simulink model "hodumaru"  (R2023a)
settings: Solver=VariableStepAuto  StartTime=0.0  StopTime=10.0  RelTol=1e-3
undefined symbols (not defined in the file): _NA, Control, DFSW, DSFW, Kill, NeuralCodedData, R_EN, RC, RC_FINAL, Spike
(part 2 of 2)

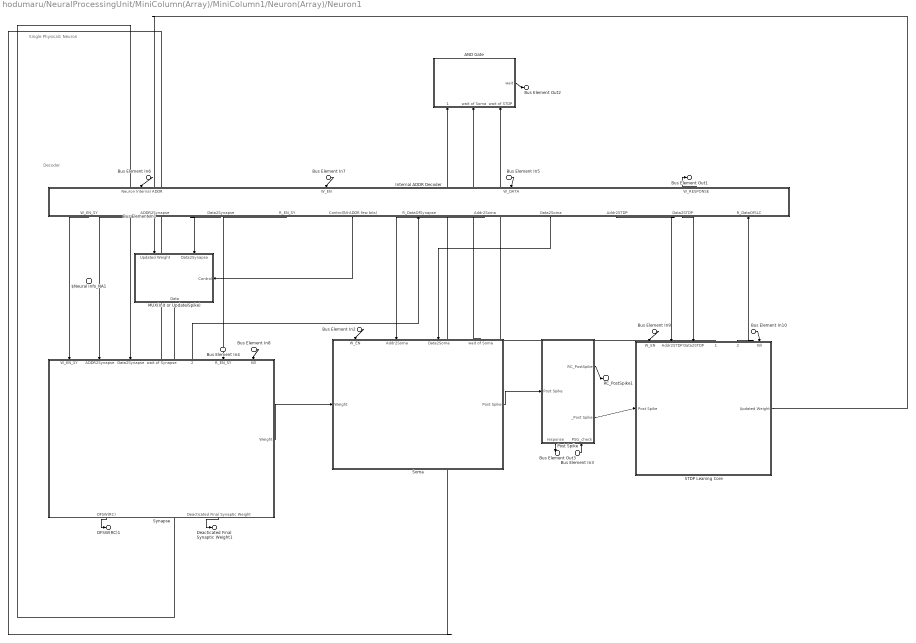
== system hodumaru/NeuralProcessingUnit/MiniColumn(Array)/MiniColumn1/Neuron(Array)/Neuron1 ==
  note: Decoder
  note: Single Physical1 Neuron
  Bus Element In3 : Inport  PortName=PSG_check
  Bus Element In1 : Inport  Port=2  PortName=#Neuron
  Bus Element In6 : Inport  Port=3  PortName=Neuron ADDR
  Bus Element In5 : Inport  Port=4  PortName=W_DATA
  Bus Element In4 : Inport  Port=5  PortName=R_EN
  Bus Element In2 : Inport  Port=6  PortName=W_EN
  Bus Element In7 : Inport  Port=6  PortName=W_EN
  Bus Element In9 : Inport  Port=6  PortName=W_EN
  Bus Element In8 : Inport  Port=7  PortName=Kill
  Bus Element In10 : Inport  Port=7  PortName=Kill
  $Neural Info_NA1 : Inport  Port=8  PortName=$Neural Info_NA
  AND Gate : Subsystem
      settings: PortSchema="{\"entries\":[{\"content\":{\"headerSize\":26,\"margin\":15,\"minimumSpacing\":25,\"sides\":[{\"content\":{},\"type\":\"ConnectorPlacement.EquallySpacedRectSide\",\"uuid\":\"ebe87d50-b34c-4144-bb21-1b9f3994f650\"},{\"content\":{\"connectorIds\":[\"Out1\"],\"side\":\"RIGHT\"},\"type\":\"ConnectorPlacement.EquallySpacedRectSide\",\"uuid\":\"40dc9e4a-9138-4a47-a8ec-83303fc3d098\"},{\"content\":{\"side\":\"TOP\"},\"type\":\"ConnectorPlacement.EquallySpacedRectSide\",\"uuid\":\"74a947e4-452e-4cf6-9818-6ec720a0f546\"},{\"content\":{\"connectorIds\":[\"In1\",\"In2\",\"In3\"],\"side\":\"BOTTOM\"},\"type\":\"ConnectorPlacement.EquallySpacedRectSide\",\"uuid\":\"c5edbbff-3ec9-45d1-a6e5-9e984b0ebe73\"}]},\"type\":\"ConnectorPlacement.EquallySpacedConnector\",\"uuid\":\"10440d1f-8be4-47e4-a65a-b886e6188624\"}],\"packageUris\":[\"http://schema.mathworks.com/mf0/Connector/R2020b\"],\"version\":\"1.0\"}"
  Internal ADDR Decoder : Subsystem
      settings: PortSchema="{\"entries\":[{\"content\":{\"headerSize\":26,\"margin\":15,\"minimumSpacing\":25,\"sides\":[{\"content\":{},\"type\":\"ConnectorPlacement.EquallySpacedRectSide\",\"uuid\":\"ebe87d50-b34c-4144-bb21-1b9f3994f650\"},{\"content\":{\"side\":\"RIGHT\"},\"type\":\"ConnectorPlacement.EquallySpacedRectSide\",\"uuid\":\"40dc9e4a-9138-4a47-a8ec-83303fc3d098\"},{\"content\":{\"connectorIds\":[\"In3\",\"In4\",\"In5\",\"Out3\"],\"side\":\"TOP\"},\"type\":\"ConnectorPlacement.EquallySpacedRectSide\",\"uuid\":\"74a947e4-452e-4cf6-9818-6ec720a0f546\"},{\"content\":{\"connectorIds\":[\"Out1\",\"Out2\",\"Out7\",\"Out4\",\"Out5\",\"In1\",\"Out6\",\"Out9\",\"Out8\",\"Out10\",\"In2\"],\"side\":\"BOTTOM\"},\"type\":\"ConnectorPlacement.EquallySpacedRectSide\",\"uuid\":\"fe67068d-9de4-4d22-acd2-463b28a86914\"}]},\"type\":\"ConnectorPlacement.EquallySpacedConnector\",\"uuid\":\"10440d1f-8be4-47e4-a65a-b886e6188624\"}],\"packageUris\":[\"http://schema.mathworks.com/mf0/Connector/R2020b\"],\"version\":\"1.0\"}"
  MUX(Init or Update/Spike) : Subsystem
      settings: PortSchema="{\"entries\":[{\"content\":{\"headerSize\":26,\"margin\":15,\"minimumSpacing\":25,\"sides\":[{\"content\":{},\"type\":\"ConnectorPlacement.EquallySpacedRectSide\",\"uuid\":\"ebe87d50-b34c-4144-bb21-1b9f3994f650\"},{\"content\":{\"connectorIds\":[\"In1\"],\"side\":\"RIGHT\"},\"type\":\"ConnectorPlacement.EquallySpacedRectSide\",\"uuid\":\"40dc9e4a-9138-4a47-a8ec-83303fc3d098\"},{\"content\":{\"connectorIds\":[\"In2\",\"In3\"],\"side\":\"TOP\"},\"type\":\"ConnectorPlacement.EquallySpacedRectSide\",\"uuid\":\"74a947e4-452e-4cf6-9818-6ec720a0f546\"},{\"content\":{\"connectorIds\":[\"Out1\"],\"side\":\"BOTTOM\"},\"type\":\"ConnectorPlacement.EquallySpacedRectSide\",\"uuid\":\"02f4fd3e-9a7d-4827-bd38-0642fed45587\"}]},\"type\":\"ConnectorPlacement.EquallySpacedConnector\",\"uuid\":\"10440d1f-8be4-47e4-a65a-b886e6188624\"}],\"packageUris\":[\"http://schema.mathworks.com/mf0/Connector/R2020b\"],\"version\":\"1.0\"}"
  Post Spike : Subsystem
      settings: PortSchema="{\"entries\":[{\"content\":{\"headerSize\":26,\"margin\":15,\"minimumSpacing\":25,\"sides\":[{\"content\":{\"connectorIds\":[\"In2\"]},\"type\":\"ConnectorPlacement.EquallySpacedRectSide\",\"uuid\":\"31e20200-2cb1-4382-9155-e0d85eeb6756\"},{\"content\":{\"connectorIds\":[\"Out2\",\"Out3\"],\"side\":\"RIGHT\"},\"type\":\"ConnectorPlacement.EquallySpacedRectSide\",\"uuid\":\"e7a9e024-b9ad-4463-a43b-85143ff39b21\"},{\"content\":{\"side\":\"TOP\"},\"type\":\"ConnectorPlacement.EquallySpacedRectSide\",\"uuid\":\"8c8eb66f-8faf-4222-8ab7-6c33983befa5\"},{\"content\":{\"connectorIds\":[\"Out1\",\"In1\"],\"side\":\"BOTTOM\"},\"type\":\"ConnectorPlacement.EquallySpacedRectSide\",\"uuid\":\"e8737092-59e1-4792-866d-bcd78d7addfa\"}]},\"type\":\"ConnectorPlacement.EquallySpacedConnector\",\"uuid\":\"7102759c-7f33-40ec-8288-a87a26b0547f\"}],\"packageUris\":[\"http://schema.mathworks.com/mf0/Connector/R2020b\"],\"version\":\"1.0\"}"
  STDP Leaning Core : Subsystem
      settings: PortSchema="{\"entries\":[{\"content\":{\"headerSize\":26,\"margin\":15,\"minimumSpacing\":25,\"sides\":[{\"content\":{\"connectorIds\":[\"In5\"]},\"type\":\"ConnectorPlacement.EquallySpacedRectSide\",\"uuid\":\"08b5c2e0-5e4b-4108-9213-5cb3cfbc2fc7\"},{\"content\":{\"connectorIds\":[\"Out3\"],\"side\":\"RIGHT\"},\"type\":\"ConnectorPlacement.EquallySpacedRectSide\",\"uuid\":\"cef344b6-f3e5-417a-912f-da0044eb54ca\"},{\"content\":{\"connectorIds\":[\"In1\",\"In2\",\"In3\",\"Out1\",\"Out2\",\"In4\"],\"side\":\"TOP\"},\"type\":\"ConnectorPlacement.EquallySpacedRectSide\",\"uuid\":\"0b83641f-e918-4d2c-8db0-09bb563129af\"}]},\"type\":\"ConnectorPlacement.EquallySpacedConnector\",\"uuid\":\"45bfd962-fc80-412c-925f-742c48c6b5c0\"}],\"packageUris\":[\"http://schema.mathworks.com/mf0/Connector/R2020b\"],\"version\":\"1.0\"}"
  Soma : Subsystem
      settings: PortSchema="{\"entries\":[{\"content\":{\"headerSize\":26,\"margin\":15,\"minimumSpacing\":25,\"sides\":[{\"content\":{\"connectorIds\":[\"In4\"]},\"type\":\"ConnectorPlacement.EquallySpacedRectSide\",\"uuid\":\"08b5c2e0-5e4b-4108-9213-5cb3cfbc2fc7\"},{\"content\":{\"connectorIds\":[\"Out2\"],\"side\":\"RIGHT\"},\"type\":\"ConnectorPlacement.EquallySpacedRectSide\",\"uuid\":\"cef344b6-f3e5-417a-912f-da0044eb54ca\"},{\"content\":{\"connectorIds\":[\"In1\",\"In2\",\"In3\",\"Out1\"],\"side\":\"TOP\"},\"type\":\"ConnectorPlacement.EquallySpacedRectSide\",\"uuid\":\"0b83641f-e918-4d2c-8db0-09bb563129af\"}]},\"type\":\"ConnectorPlacement.EquallySpacedConnector\",\"uuid\":\"45bfd962-fc80-412c-925f-742c48c6b5c0\"}],\"packageUris\":[\"http://schema.mathworks.com/mf0/Connector/R2020b\"],\"version\":\"1.0\"}"
  Synapse : Subsystem
      settings: PortSchema="{\"entries\":[{\"content\":{\"headerSize\":26,\"margin\":15,\"minimumSpacing\":25,\"sides\":[{\"content\":{},\"type\":\"ConnectorPlacement.EquallySpacedRectSide\",\"uuid\":\"08b5c2e0-5e4b-4108-9213-5cb3cfbc2fc7\"},{\"content\":{\"connectorIds\":[\"Out3\"],\"side\":\"RIGHT\"},\"type\":\"ConnectorPlacement.EquallySpacedRectSide\",\"uuid\":\"cef344b6-f3e5-417a-912f-da0044eb54ca\"},{\"content\":{\"connectorIds\":[\"In1\",\"In2\",\"In3\",\"Out1\",\"Out2\",\"In4\",\"In5\"],\"side\":\"TOP\"},\"type\":\"ConnectorPlacement.EquallySpacedRectSide\",\"uuid\":\"0b83641f-e918-4d2c-8db0-09bb563129af\"},{\"content\":{\"connectorIds\":[\"Out5\",\"Out4\"],\"side\":\"BOTTOM\"},\"type\":\"ConnectorPlacement.EquallySpacedRectSide\",\"uuid\":\"115d5a97-31cb-4c10-ac03-233646a622a9\"}]},\"type\":\"ConnectorPlacement.EquallySpacedConnector\",\"uuid\":\"45bfd962-fc80-412c-925f-742c48c6b5c0\"}],\"packageUris\":[\"http://schema.mathworks.com/mf0/Connector/R2020b\"],\"version\":\"1.0\"}"
  Bus Element Out3 : Outport  PortName=response
  Bus Element Out2 : Outport  Port=2  PortName=wait
  Bus Element Out1 : Outport  Port=3  PortName=W_RESPONSE
  RC_PostSpike1 : Outport  Port=4  PortName=RC_PostSpike
  Deacticated Final Synaptic Weight1 : Outport  Port=5  PortName=Deacticated Final Synaptic Weight
  DFSW(RC)1 : Outport  Port=6  PortName=DFSW(RC)
  wires:
  Synapse/5(DFSW(RC)) -> DFSW(RC)1/1
  STDP Leaning Core/3(Updated Weight) -> MUX(Init or Update/Spike)/2(Updated Weight)
  Synapse/3(Weight) -> Soma/4(Weight)
  Soma/2(Post Spike) -> Post Spike/2(Post Spike)
  Post Spike/3(_Post Spike) -> STDP Leaning Core/5(Post Spike)
  Synapse/4(Deacticated Final Synaptic Weight) -> Deacticated Final Synaptic Weight1/1
  Post Spike/2(RC_PostSpike) -> RC_PostSpike1/1
  Bus Element In2/1 -> Soma/1(W_EN)
  Bus Element In6/1 -> Internal ADDR Decoder/3(Neuron Internal ADDR)
  Internal ADDR Decoder/7(Data2Synapse) -> MUX(Init or Update/Spike)/3(Data2Synapse)
  Internal ADDR Decoder/9(Data2Soma) -> Soma/3(Data2Soma)
  Internal ADDR Decoder/10(Data2STDP) -> STDP Leaning Core/3(Data2STDP)
  Bus Element In5/1 -> Internal ADDR Decoder/5(W_DATA)
  Bus Element In7/1 -> Internal ADDR Decoder/4(W_EN)
  Internal ADDR Decoder/3(W_RESPONSE) -> Bus Element Out1/1
  Internal ADDR Decoder/2(ADDR2Synapse) -> Synapse/2(ADDR2Synapse)
  Internal ADDR Decoder/6(Addr2Soma) -> Soma/2(Addr2Soma)
  Synapse/2(R_DataOfSynapse) -> Internal ADDR Decoder/1(R_DataOfSynapse)
  STDP Leaning Core/2(R_DataOfSLC) -> Internal ADDR Decoder/2(R_DataOfSLC)
  MUX(Init or Update/Spike)/1(Data) -> Synapse/3(Data2Synapse)
  Bus Element In8/1 -> Synapse/5(Kill)
  Internal ADDR Decoder/5(Control(NI-ADDR few bits)) -> MUX(Init or Update/Spike)/1(Control)
  Synapse/1(wait of Synapse) -> AND Gate/1(wait of Synapse)
  Soma/1(wait of Soma) -> AND Gate/2(wait of Soma)
  STDP Leaning Core/1(wait of STDP) -> AND Gate/3(wait of STDP)
  AND Gate/1(wait) -> Bus Element Out2/1
  Internal ADDR Decoder/8(Addr2STDP) -> STDP Leaning Core/2(Addr2STDP)
  Bus Element In9/1 -> STDP Leaning Core/1(W_EN)
  Bus Element In10/1 -> STDP Leaning Core/4(Kill)
  Internal ADDR Decoder/1(W_EN_SY) -> Synapse/1(W_EN_SY)
  Internal ADDR Decoder/4(R_EN_SY) -> Synapse/4(R_EN_SY)
  Post Spike/1(response) -> Bus Element Out3/1
  Bus Element In3/1 -> Post Spike/1(PSG_check)

== system hodumaru/NeuralProcessingUnit/MiniColumn(Array)/MiniColumn2/Neuron(Array)/Neuron Init ==
  Bus Element In1 : Inport  PortName=$Neural Info_NA
  Bus Element Out3 : Outport  PortName=STDP Curve_Init
  Bus Element Out2 : Outport  Port=2  PortName=Soma Type_Init
  Bus Element Out1 : Outport  Port=3  PortName=Synapse_Init

== system hodumaru/NeuralProcessingUnit/MiniColumn(Array)/MiniColumn2/Neuron(Array)/Post Spike ==
  Bus Element In1 : Inport  PortName=Post Spike
  Bus Element Out1 : Outport  PortName=RC_PostSpike
  Bus Element Out2 : Outport  Port=2  PortName=OutBus

== system hodumaru/NeuralProcessingUnit/MiniColumn(Array)/MiniColumn2/Neuron(Array)/STDP Leaning Core ==
  Bus Element In3 : Inport  PortName=Post Spike
  Bus Element In1 : Inport  Port=2  PortName=STDP Curve_Init
  Bus Element In2 : Inport  Port=3  PortName=External Spike
  STDP Curve LUT : Subsystem
      settings: PortSchema="{\"entries\":[{\"content\":{\"headerSize\":26,\"margin\":15,\"minimumSpacing\":25,\"sides\":[{\"content\":{\"connectorIds\":[\"In1\"]},\"type\":\"ConnectorPlacement.EquallySpacedRectSide\",\"uuid\":\"31e20200-2cb1-4382-9155-e0d85eeb6756\"},{\"content\":{\"connectorIds\":[\"Out1\"],\"side\":\"RIGHT\"},\"type\":\"ConnectorPlacement.EquallySpacedRectSide\",\"uuid\":\"e7a9e024-b9ad-4463-a43b-85143ff39b21\"},{\"content\":{\"connectorIds\":[\"In2\"],\"side\":\"TOP\"},\"type\":\"ConnectorPlacement.EquallySpacedRectSide\",\"uuid\":\"8c8eb66f-8faf-4222-8ab7-6c33983befa5\"}]},\"type\":\"ConnectorPlacement.EquallySpacedConnector\",\"uuid\":\"7102759c-7f33-40ec-8288-a87a26b0547f\"}],\"packageUris\":[\"http://schema.mathworks.com/mf0/Connector/R2020b\"],\"version\":\"1.0\"}"
  Time Difference checker : Subsystem
      settings: PortSchema="{\"entries\":[{\"content\":{\"headerSize\":26,\"margin\":15,\"minimumSpacing\":25,\"sides\":[{\"content\":{\"connectorIds\":[\"In1\",\"In2\"]},\"type\":\"ConnectorPlacement.EquallySpacedRectSide\",\"uuid\":\"31e20200-2cb1-4382-9155-e0d85eeb6756\"},{\"content\":{\"connectorIds\":[\"Out1\"],\"side\":\"RIGHT\"},\"type\":\"ConnectorPlacement.EquallySpacedRectSide\",\"uuid\":\"e7a9e024-b9ad-4463-a43b-85143ff39b21\"},{\"content\":{\"side\":\"TOP\"},\"type\":\"ConnectorPlacement.EquallySpacedRectSide\",\"uuid\":\"8c8eb66f-8faf-4222-8ab7-6c33983befa5\"}]},\"type\":\"ConnectorPlacement.EquallySpacedConnector\",\"uuid\":\"7102759c-7f33-40ec-8288-a87a26b0547f\"}],\"packageUris\":[\"http://schema.mathworks.com/mf0/Connector/R2020b\"],\"version\":\"1.0\"}"
  Bus Element Out2 : Outport  PortName=Updated Weight
  wires:
  Bus Element In3/1 -> Time Difference checker/1(Post Spike)
  Bus Element In2/1 -> Time Difference checker/2(External Spike)
  Bus Element In1/1 -> STDP Curve LUT/2(STDP Curve_Init)
  Time Difference checker/1(Time Difference) -> STDP Curve LUT/1(Time Difference)
  STDP Curve LUT/1(Updated Weight) -> Bus Element Out2/1

== system hodumaru/NeuralProcessingUnit/MiniColumn(Array)/MiniColumn2/Neuron(Array)/Soma ==
  Bus Element In2 : Inport  PortName=Soma Type_Init
  Bus Element In1 : Inport  Port=2  PortName=Weighted Spike
  Membrane Potential Computing Unit : Subsystem
      settings: PortSchema="{\"entries\":[{\"content\":{\"headerSize\":26,\"margin\":15,\"minimumSpacing\":25,\"sides\":[{\"content\":{\"connectorIds\":[\"In1\"]},\"type\":\"ConnectorPlacement.EquallySpacedRectSide\",\"uuid\":\"08b5c2e0-5e4b-4108-9213-5cb3cfbc2fc7\"},{\"content\":{\"connectorIds\":[\"Out1\"],\"side\":\"RIGHT\"},\"type\":\"ConnectorPlacement.EquallySpacedRectSide\",\"uuid\":\"cef344b6-f3e5-417a-912f-da0044eb54ca\"},{\"content\":{\"side\":\"TOP\"},\"type\":\"ConnectorPlacement.EquallySpacedRectSide\",\"uuid\":\"0b83641f-e918-4d2c-8db0-09bb563129af\"}]},\"type\":\"ConnectorPlacement.EquallySpacedConnector\",\"uuid\":\"45bfd962-fc80-412c-925f-742c48c6b5c0\"}],\"packageUris\":[\"http://schema.mathworks.com/mf0/Connector/R2020b\"],\"version\":\"1.0\"}"
  Bus Element Out1 : Outport  PortName=Post Spike
  wires:
  Bus Element In1/1 -> Membrane Potential Computing Unit/1(Weighted Spike)
  Membrane Potential Computing Unit/1(Post Spike) -> Bus Element Out1/1

== system hodumaru/NeuralProcessingUnit/MiniColumn(Array)/MiniColumn2/Neuron(Array)/Synapse ==
  Bus Element In4 : Inport  PortName=External Spike2
  Bus Element In3 : Inport  Port=2  PortName=Synapse_Init
  Bus Element In2 : Inport  Port=3  PortName=Updated Weight
  Bus Element In1 : Inport  Port=4  PortName=External Spike
  Weight Compute unit : Subsystem
      settings: PortSchema="{\"entries\":[{\"content\":{\"headerSize\":26,\"margin\":15,\"minimumSpacing\":25,\"sides\":[{\"content\":{\"connectorIds\":[\"In1\"]},\"type\":\"ConnectorPlacement.EquallySpacedRectSide\",\"uuid\":\"08b5c2e0-5e4b-4108-9213-5cb3cfbc2fc7\"},{\"content\":{\"connectorIds\":[\"Out1\"],\"side\":\"RIGHT\"},\"type\":\"ConnectorPlacement.EquallySpacedRectSide\",\"uuid\":\"cef344b6-f3e5-417a-912f-da0044eb54ca\"},{\"content\":{\"side\":\"TOP\"},\"type\":\"ConnectorPlacement.EquallySpacedRectSide\",\"uuid\":\"0b83641f-e918-4d2c-8db0-09bb563129af\"}]},\"type\":\"ConnectorPlacement.EquallySpacedConnector\",\"uuid\":\"45bfd962-fc80-412c-925f-742c48c6b5c0\"}],\"packageUris\":[\"http://schema.mathworks.com/mf0/Connector/R2020b\"],\"version\":\"1.0\"}"
  Bus Element Out1 : Outport  PortName=Weighted Spike
  Bus Element Out2 : Outport  Port=2  PortName=Deacticated Final Synaptic Weight
  Bus Element Out3 : Outport  Port=3  PortName=DFSW(RC)
  wires:
  Bus Element In1/1 -> Weight Compute unit/1(External Spike)
  Weight Compute unit/1(Weighted Spike) -> Bus Element Out1/1

== system hodumaru/NeuralProcessingUnit/MiniColumn(Array)/MiniColumn1/Neuron(Array)/Neuron1/AND Gate ==
  Bus Element In1 : Inport  PortName=wait of Synapse
  Bus Element In2 : Inport  Port=2  PortName=wait of Soma
  Bus Element In3 : Inport  Port=3  PortName=wait of STDP
  Bus Element Out1 : Outport  PortName=wait

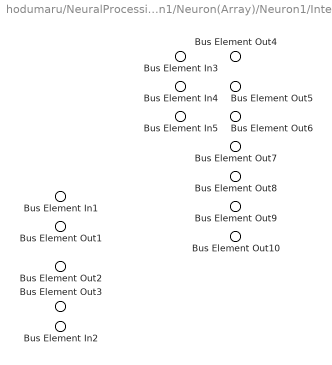
== system hodumaru/NeuralProcessingUnit/MiniColumn(Array)/MiniColumn1/Neuron(Array)/Neuron1/Internal ADDR Decoder ==
  Bus Element In4 : Inport  PortName=R_DataOfSynapse
  Bus Element In5 : Inport  Port=2  PortName=R_DataOfSLC
  Bus Element In1 : Inport  Port=3  PortName=Neuron Internal ADDR
  Bus Element In3 : Inport  Port=4  PortName=W_EN
  Bus Element In2 : Inport  Port=5  PortName=W_DATA
  Bus Element Out9 : Outport  PortName=W_EN_SY
  Bus Element Out5 : Outport  Port=2  PortName=ADDR2Synapse
  Bus Element Out4 : Outport  Port=3  PortName=W_RESPONSE
  Bus Element Out10 : Outport  Port=4  PortName=R_EN_SY
  Bus Element Out7 : Outport  Port=5  PortName=Control(NI-ADDR few bits)
  Bus Element Out6 : Outport  Port=6  PortName=Addr2Soma
  Bus Element Out1 : Outport  Port=7  PortName=Data2Synapse
  Bus Element Out8 : Outport  Port=8  PortName=Addr2STDP
  Bus Element Out2 : Outport  Port=9  PortName=Data2Soma
  Bus Element Out3 : Outport  Port=10  PortName=Data2STDP

== system hodumaru/NeuralProcessingUnit/MiniColumn(Array)/MiniColumn1/Neuron(Array)/Neuron1/MUX(Init or Update//Spike) ==
  Bus Element In3 : Inport  PortName=Control
  Bus Element In1 : Inport  Port=2  PortName=Updated Weight
  Bus Element In2 : Inport  Port=3  PortName=Data2Synapse
  Bus Element Out1 : Outport  PortName=Data

== system hodumaru/NeuralProcessingUnit/MiniColumn(Array)/MiniColumn1/Neuron(Array)/Neuron1/Post Spike ==
  Bus Element In2 : Inport  PortName=PSG_check
  Bus Element In1 : Inport  Port=2  PortName=Post Spike
  Bus Element Out3 : Outport  PortName=response
  Bus Element Out1 : Outport  Port=2  PortName=RC_PostSpike
  Bus Element Out2 : Outport  Port=3  PortName=_Post Spike

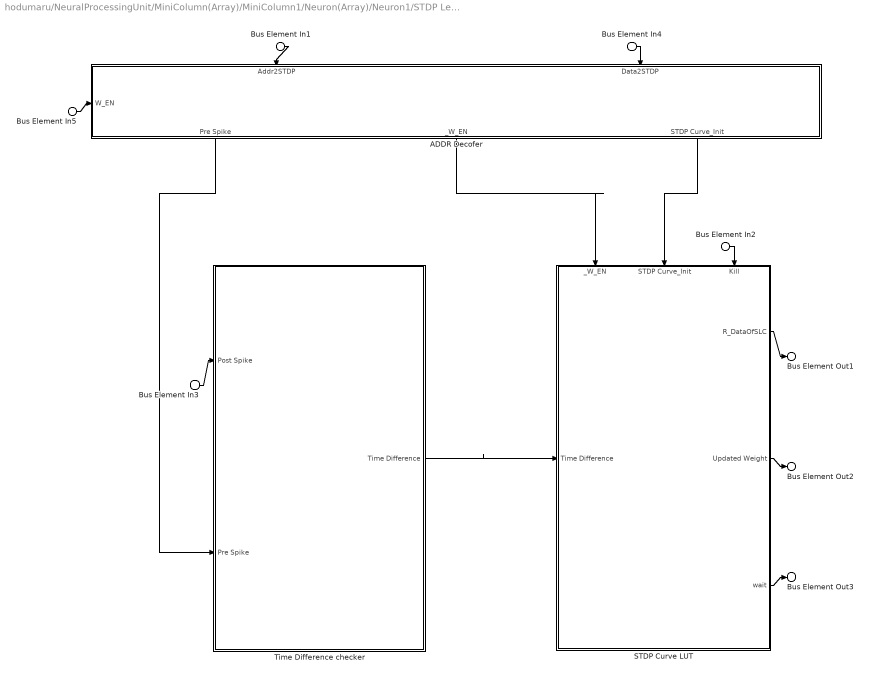
== system hodumaru/NeuralProcessingUnit/MiniColumn(Array)/MiniColumn1/Neuron(Array)/Neuron1/STDP Leaning Core ==
  Bus Element In5 : Inport  PortName=W_EN
  Bus Element In1 : Inport  Port=2  PortName=Addr2STDP
  Bus Element In4 : Inport  Port=3  PortName=Data2STDP
  Bus Element In2 : Inport  Port=4  PortName=Kill
  Bus Element In3 : Inport  Port=5  PortName=Post Spike
  ADDR Decofer : Subsystem
      settings: PortSchema="{\"entries\":[{\"content\":{\"headerSize\":26,\"margin\":15,\"minimumSpacing\":25,\"sides\":[{\"content\":{\"connectorIds\":[\"In1\"]},\"type\":\"ConnectorPlacement.EquallySpacedRectSide\",\"uuid\":\"ebe87d50-b34c-4144-bb21-1b9f3994f650\"},{\"content\":{\"side\":\"RIGHT\"},\"type\":\"ConnectorPlacement.EquallySpacedRectSide\",\"uuid\":\"40dc9e4a-9138-4a47-a8ec-83303fc3d098\"},{\"content\":{\"connectorIds\":[\"In2\",\"In3\"],\"side\":\"TOP\"},\"type\":\"ConnectorPlacement.EquallySpacedRectSide\",\"uuid\":\"74a947e4-452e-4cf6-9818-6ec720a0f546\"},{\"content\":{\"connectorIds\":[\"Out1\",\"Out2\",\"Out3\"],\"side\":\"BOTTOM\"},\"type\":\"ConnectorPlacement.EquallySpacedRectSide\",\"uuid\":\"ec563be9-e838-4afa-83e3-9f80d5479a26\"}]},\"type\":\"ConnectorPlacement.EquallySpacedConnector\",\"uuid\":\"10440d1f-8be4-47e4-a65a-b886e6188624\"}],\"packageUris\":[\"http://schema.mathworks.com/mf0/Connector/R2020b\"],\"version\":\"1.0\"}"
  STDP Curve LUT : Subsystem
      settings: PortSchema="{\"entries\":[{\"content\":{\"headerSize\":26,\"margin\":15,\"minimumSpacing\":25,\"sides\":[{\"content\":{\"connectorIds\":[\"In2\"]},\"type\":\"ConnectorPlacement.EquallySpacedRectSide\",\"uuid\":\"31e20200-2cb1-4382-9155-e0d85eeb6756\"},{\"content\":{\"connectorIds\":[\"Out1\",\"Out3\",\"Out2\"],\"side\":\"RIGHT\"},\"type\":\"ConnectorPlacement.EquallySpacedRectSide\",\"uuid\":\"e7a9e024-b9ad-4463-a43b-85143ff39b21\"},{\"content\":{\"connectorIds\":[\"In1\",\"In4\",\"In3\"],\"side\":\"TOP\"},\"type\":\"ConnectorPlacement.EquallySpacedRectSide\",\"uuid\":\"8c8eb66f-8faf-4222-8ab7-6c33983befa5\"}]},\"type\":\"ConnectorPlacement.EquallySpacedConnector\",\"uuid\":\"7102759c-7f33-40ec-8288-a87a26b0547f\"}],\"packageUris\":[\"http://schema.mathworks.com/mf0/Connector/R2020b\"],\"version\":\"1.0\"}"
  Time Difference checker : Subsystem
      settings: PortSchema="{\"entries\":[{\"content\":{\"headerSize\":26,\"margin\":15,\"minimumSpacing\":25,\"sides\":[{\"content\":{\"connectorIds\":[\"In1\",\"In2\"]},\"type\":\"ConnectorPlacement.EquallySpacedRectSide\",\"uuid\":\"31e20200-2cb1-4382-9155-e0d85eeb6756\"},{\"content\":{\"connectorIds\":[\"Out1\"],\"side\":\"RIGHT\"},\"type\":\"ConnectorPlacement.EquallySpacedRectSide\",\"uuid\":\"e7a9e024-b9ad-4463-a43b-85143ff39b21\"},{\"content\":{\"side\":\"TOP\"},\"type\":\"ConnectorPlacement.EquallySpacedRectSide\",\"uuid\":\"8c8eb66f-8faf-4222-8ab7-6c33983befa5\"}]},\"type\":\"ConnectorPlacement.EquallySpacedConnector\",\"uuid\":\"7102759c-7f33-40ec-8288-a87a26b0547f\"}],\"packageUris\":[\"http://schema.mathworks.com/mf0/Connector/R2020b\"],\"version\":\"1.0\"}"
  Bus Element Out3 : Outport  PortName=wait of STDP
  Bus Element Out1 : Outport  Port=2  PortName=R_DataOfSLC
  Bus Element Out2 : Outport  Port=3  PortName=Updated Weight
  wires:
  Bus Element In3/1 -> Time Difference checker/1(Post Spike)
  ADDR Decofer/3(STDP Curve_Init) -> STDP Curve LUT/4(STDP Curve_Init)
  Time Difference checker/1(Time Difference) -> STDP Curve LUT/2(Time Difference)
  STDP Curve LUT/3(Updated Weight) -> Bus Element Out2/1
  STDP Curve LUT/2(wait) -> Bus Element Out3/1
  Bus Element In1/1 -> ADDR Decofer/2(Addr2STDP)
  Bus Element In4/1 -> ADDR Decofer/3(Data2STDP)
  Bus Element In5/1 -> ADDR Decofer/1(W_EN)
  ADDR Decofer/1(Pre Spike) -> Time Difference checker/2(Pre Spike)
  ADDR Decofer/2(_W_EN) -> STDP Curve LUT/1(_W_EN)
  Bus Element In2/1 -> STDP Curve LUT/3(Kill)
  STDP Curve LUT/1(R_DataOfSLC) -> Bus Element Out1/1

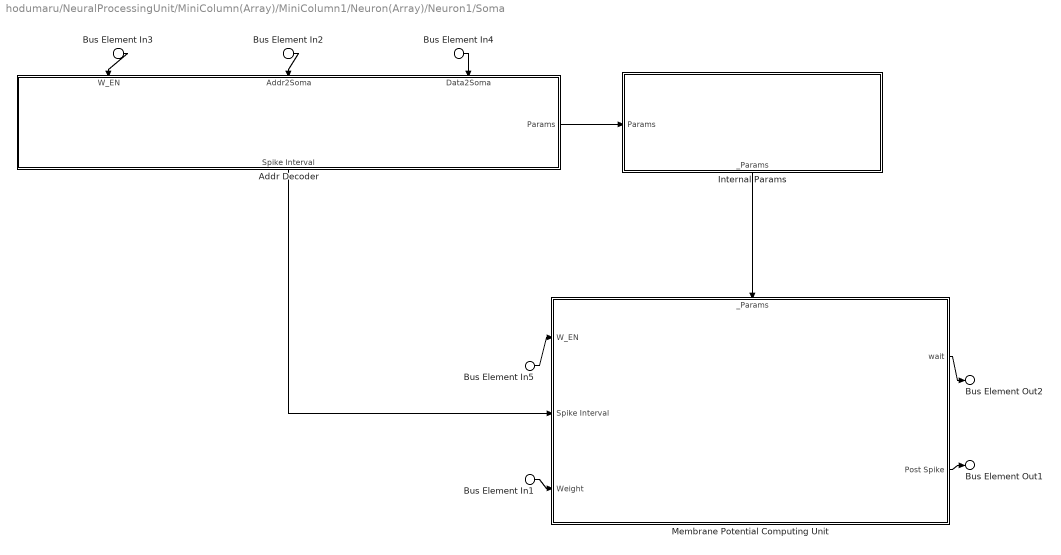
== system hodumaru/NeuralProcessingUnit/MiniColumn(Array)/MiniColumn1/Neuron(Array)/Neuron1/Soma ==
  Bus Element In3 : Inport  PortName=W_EN
  Bus Element In5 : Inport  PortName=W_EN
  Bus Element In2 : Inport  Port=2  PortName=Addr2Soma
  Bus Element In4 : Inport  Port=3  PortName=Data2Soma
  Bus Element In1 : Inport  Port=4  PortName=Weight
  Addr Decoder : Subsystem
      settings: PortSchema="{\"entries\":[{\"content\":{\"headerSize\":26,\"margin\":15,\"minimumSpacing\":25,\"sides\":[{\"content\":{},\"type\":\"ConnectorPlacement.EquallySpacedRectSide\",\"uuid\":\"ebe87d50-b34c-4144-bb21-1b9f3994f650\"},{\"content\":{\"connectorIds\":[\"Out2\"],\"side\":\"RIGHT\"},\"type\":\"ConnectorPlacement.EquallySpacedRectSide\",\"uuid\":\"40dc9e4a-9138-4a47-a8ec-83303fc3d098\"},{\"content\":{\"connectorIds\":[\"In1\",\"In2\",\"In3\"],\"side\":\"TOP\"},\"type\":\"ConnectorPlacement.EquallySpacedRectSide\",\"uuid\":\"74a947e4-452e-4cf6-9818-6ec720a0f546\"},{\"content\":{\"connectorIds\":[\"Out1\"],\"side\":\"BOTTOM\"},\"type\":\"ConnectorPlacement.EquallySpacedRectSide\",\"uuid\":\"271d9355-769d-4bff-8bc1-4135afb0f0d9\"}]},\"type\":\"ConnectorPlacement.EquallySpacedConnector\",\"uuid\":\"10440d1f-8be4-47e4-a65a-b886e6188624\"}],\"packageUris\":[\"http://schema.mathworks.com/mf0/Connector/R2020b\"],\"version\":\"1.0\"}"
  Internal Params : Subsystem
      settings: PortSchema="{\"entries\":[{\"content\":{\"headerSize\":26,\"margin\":15,\"minimumSpacing\":25,\"sides\":[{\"content\":{\"connectorIds\":[\"In1\"]},\"type\":\"ConnectorPlacement.EquallySpacedRectSide\",\"uuid\":\"ebe87d50-b34c-4144-bb21-1b9f3994f650\"},{\"content\":{\"side\":\"RIGHT\"},\"type\":\"ConnectorPlacement.EquallySpacedRectSide\",\"uuid\":\"40dc9e4a-9138-4a47-a8ec-83303fc3d098\"},{\"content\":{\"side\":\"TOP\"},\"type\":\"ConnectorPlacement.EquallySpacedRectSide\",\"uuid\":\"74a947e4-452e-4cf6-9818-6ec720a0f546\"},{\"content\":{\"connectorIds\":[\"Out1\"],\"side\":\"BOTTOM\"},\"type\":\"ConnectorPlacement.EquallySpacedRectSide\",\"uuid\":\"57904876-d35b-47b5-82f0-729b1bead8bf\"}]},\"type\":\"ConnectorPlacement.EquallySpacedConnector\",\"uuid\":\"10440d1f-8be4-47e4-a65a-b886e6188624\"}],\"packageUris\":[\"http://schema.mathworks.com/mf0/Connector/R2020b\"],\"version\":\"1.0\"}"
  Membrane Potential Computing Unit : Subsystem
      settings: PortSchema="{\"entries\":[{\"content\":{\"headerSize\":26,\"margin\":15,\"minimumSpacing\":25,\"sides\":[{\"content\":{\"connectorIds\":[\"In1\",\"In2\",\"In4\"]},\"type\":\"ConnectorPlacement.EquallySpacedRectSide\",\"uuid\":\"08b5c2e0-5e4b-4108-9213-5cb3cfbc2fc7\"},{\"content\":{\"connectorIds\":[\"Out1\",\"Out2\"],\"side\":\"RIGHT\"},\"type\":\"ConnectorPlacement.EquallySpacedRectSide\",\"uuid\":\"cef344b6-f3e5-417a-912f-da0044eb54ca\"},{\"content\":{\"connectorIds\":[\"In3\"],\"side\":\"TOP\"},\"type\":\"ConnectorPlacement.EquallySpacedRectSide\",\"uuid\":\"0b83641f-e918-4d2c-8db0-09bb563129af\"}]},\"type\":\"ConnectorPlacement.EquallySpacedConnector\",\"uuid\":\"45bfd962-fc80-412c-925f-742c48c6b5c0\"}],\"packageUris\":[\"http://schema.mathworks.com/mf0/Connector/R2020b\"],\"version\":\"1.0\"}"
  Bus Element Out2 : Outport  PortName=wait of Soma
  Bus Element Out1 : Outport  Port=2  PortName=Post Spike
  wires:
  Bus Element In1/1 -> Membrane Potential Computing Unit/4(Weight)
  Membrane Potential Computing Unit/2(Post Spike) -> Bus Element Out1/1
  Bus Element In2/1 -> Addr Decoder/2(Addr2Soma)
  Bus Element In4/1 -> Addr Decoder/3(Data2Soma)
  Addr Decoder/2(Params) -> Internal Params/1(Params)
  Internal Params/1(_Params) -> Membrane Potential Computing Unit/3(_Params)
  Membrane Potential Computing Unit/1(wait) -> Bus Element Out2/1
  Addr Decoder/1(Spike Interval) -> Membrane Potential Computing Unit/2(Spike Interval)
  Bus Element In3/1 -> Addr Decoder/1(W_EN)
  Bus Element In5/1 -> Membrane Potential Computing Unit/1(W_EN)

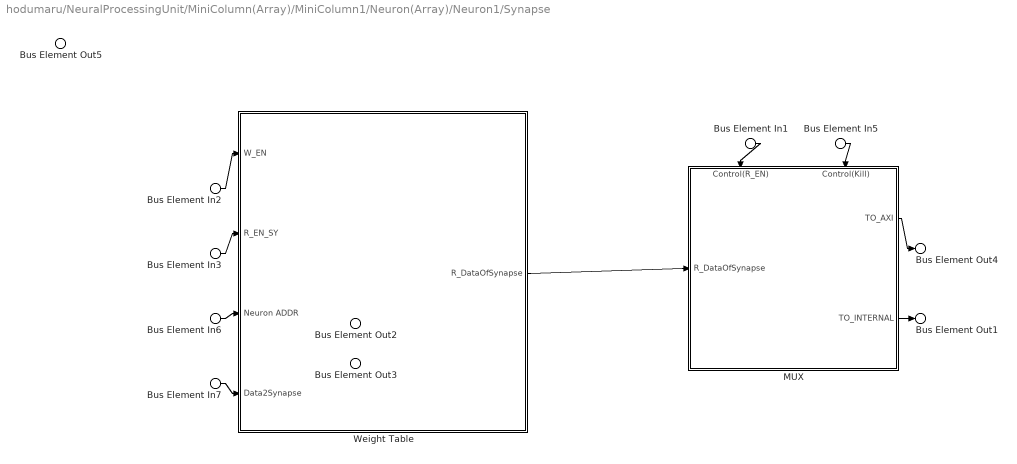
== system hodumaru/NeuralProcessingUnit/MiniColumn(Array)/MiniColumn1/Neuron(Array)/Neuron1/Synapse ==
  Bus Element In2 : Inport  PortName=W_EN_SY
  Bus Element In6 : Inport  Port=2  PortName=ADDR2Synapse
  Bus Element In7 : Inport  Port=3  PortName=Data2Synapse
  Bus Element In1 : Inport  Port=4  PortName=R_EN_SY
  Bus Element In3 : Inport  Port=4  PortName=R_EN_SY
  Bus Element In5 : Inport  Port=5  PortName=Kill
  MUX : Subsystem
      settings: PortSchema="{\"entries\":[{\"content\":{\"headerSize\":26,\"margin\":15,\"minimumSpacing\":25,\"sides\":[{\"content\":{\"connectorIds\":[\"In3\"]},\"type\":\"ConnectorPlacement.EquallySpacedRectSide\",\"uuid\":\"ebe87d50-b34c-4144-bb21-1b9f3994f650\"},{\"content\":{\"connectorIds\":[\"Out1\",\"Out2\"],\"side\":\"RIGHT\"},\"type\":\"ConnectorPlacement.EquallySpacedRectSide\",\"uuid\":\"40dc9e4a-9138-4a47-a8ec-83303fc3d098\"},{\"content\":{\"connectorIds\":[\"In1\",\"In2\"],\"side\":\"TOP\"},\"type\":\"ConnectorPlacement.EquallySpacedRectSide\",\"uuid\":\"74a947e4-452e-4cf6-9818-6ec720a0f546\"}]},\"type\":\"ConnectorPlacement.EquallySpacedConnector\",\"uuid\":\"10440d1f-8be4-47e4-a65a-b886e6188624\"}],\"packageUris\":[\"http://schema.mathworks.com/mf0/Connector/R2020b\"],\"version\":\"1.0\"}"
  Weight Table : Subsystem
      settings: PortSchema="{\"entries\":[{\"content\":{\"headerSize\":26,\"margin\":15,\"minimumSpacing\":25,\"sides\":[{\"content\":{\"connectorIds\":[\"In1\",\"In2\",\"In4\",\"In3\"]},\"type\":\"ConnectorPlacement.EquallySpacedRectSide\",\"uuid\":\"ebe87d50-b34c-4144-bb21-1b9f3994f650\"},{\"content\":{\"connectorIds\":[\"Out1\"],\"side\":\"RIGHT\"},\"type\":\"ConnectorPlacement.EquallySpacedRectSide\",\"uuid\":\"40dc9e4a-9138-4a47-a8ec-83303fc3d098\"},{\"content\":{\"side\":\"TOP\"},\"type\":\"ConnectorPlacement.EquallySpacedRectSide\",\"uuid\":\"74a947e4-452e-4cf6-9818-6ec720a0f546\"}]},\"type\":\"ConnectorPlacement.EquallySpacedConnector\",\"uuid\":\"10440d1f-8be4-47e4-a65a-b886e6188624\"}],\"packageUris\":[\"http://schema.mathworks.com/mf0/Connector/R2020b\"],\"version\":\"1.0\"}"
  Bus Element Out5 : Outport  PortName=wait of Synapse
  Bus Element Out4 : Outport  Port=2  PortName=R_DataOfSynapse
  Bus Element Out1 : Outport  Port=3  PortName=Weight
  Bus Element Out2 : Outport  Port=4  PortName=Deacticated Final Synaptic Weight
  Bus Element Out3 : Outport  Port=5  PortName=DFSW(RC)
  wires:
  Weight Table/1(R_DataOfSynapse) -> MUX/3(R_DataOfSynapse)
  MUX/1(TO_AXI) -> Bus Element Out4/1
  Bus Element In7/1 -> Weight Table/3(Data2Synapse)
  MUX/2(TO_INTERNAL) -> Bus Element Out1/1
  Bus Element In5/1 -> MUX/2(Control(Kill))
  Bus Element In1/1 -> MUX/1(Control(R_EN))
  Bus Element In2/1 -> Weight Table/1(W_EN)
  Bus Element In3/1 -> Weight Table/2(R_EN_SY)
  Bus Element In6/1 -> Weight Table/4(Neuron ADDR)

== system hodumaru/NeuralProcessingUnit/MiniColumn(Array)/MiniColumn2/Neuron(Array)/STDP Leaning Core/STDP Curve LUT ==
  Bus Element In2 : Inport  PortName=Time Difference
  Bus Element In1 : Inport  Port=2  PortName=STDP Curve_Init
  Bus Element Out1 : Outport  PortName=Updated Weight

== system hodumaru/NeuralProcessingUnit/MiniColumn(Array)/MiniColumn2/Neuron(Array)/STDP Leaning Core/Time Difference checker ==
  Bus Element In1 : Inport  PortName=Post Spike
  Bus Element In2 : Inport  Port=2  PortName=External Spike
  Bus Element Out1 : Outport  PortName=Time Difference

== system hodumaru/NeuralProcessingUnit/MiniColumn(Array)/MiniColumn2/Neuron(Array)/Soma/Membrane Potential Computing Unit ==
  Bus Element In1 : Inport  PortName=Weighted Spike
  Bus Element Out1 : Outport  PortName=Post Spike

== system hodumaru/NeuralProcessingUnit/MiniColumn(Array)/MiniColumn2/Neuron(Array)/Synapse/Weight Compute unit ==
  Bus Element In1 : Inport  PortName=External Spike
  Bus Element Out1 : Outport  PortName=Weighted Spike

== system hodumaru/NeuralProcessingUnit/MiniColumn(Array)/MiniColumn1/Neuron(Array)/Neuron1/STDP Leaning Core/ADDR Decofer ==
  Bus Element In3 : Inport  PortName=W_EN
  Bus Element In1 : Inport  Port=2  PortName=Addr2STDP
  Bus Element In2 : Inport  Port=3  PortName=Data2STDP
  Bus Element Out2 : Outport  PortName=Pre Spike
  Bus Element Out3 : Outport  Port=2  PortName=_W_EN
  Bus Element Out1 : Outport  Port=3  PortName=STDP Curve_Init

== system hodumaru/NeuralProcessingUnit/MiniColumn(Array)/MiniColumn1/Neuron(Array)/Neuron1/STDP Leaning Core/STDP Curve LUT ==
  Bus Element In3 : Inport  PortName=_W_EN
  Bus Element In2 : Inport  Port=2  PortName=Time Difference
  Bus Element In4 : Inport  Port=3  PortName=Kill
  Bus Element In1 : Inport  Port=4  PortName=STDP Curve_Init
  Bus Element Out3 : Outport  PortName=R_DataOfSLC
  Bus Element Out2 : Outport  Port=2  PortName=wait
  Bus Element Out1 : Outport  Port=3  PortName=Updated Weight

== system hodumaru/NeuralProcessingUnit/MiniColumn(Array)/MiniColumn1/Neuron(Array)/Neuron1/STDP Leaning Core/Time Difference checker ==
  Bus Element In1 : Inport  PortName=Post Spike
  Bus Element In3 : Inport  Port=2  PortName=Pre Spike
  Bus Element Out1 : Outport  PortName=Time Difference

== system hodumaru/NeuralProcessingUnit/MiniColumn(Array)/MiniColumn1/Neuron(Array)/Neuron1/Soma/Addr Decoder ==
  Bus Element In3 : Inport  PortName=W_EN
  Bus Element In1 : Inport  Port=2  PortName=Addr2Soma
  Bus Element In2 : Inport  Port=3  PortName=Data2Soma
  Bus Element Out2 : Outport  PortName=Spike Interval
  Bus Element Out1 : Outport  Port=2  PortName=Params

== system hodumaru/NeuralProcessingUnit/MiniColumn(Array)/MiniColumn1/Neuron(Array)/Neuron1/Soma/Internal Params ==
  Bus Element In1 : Inport  PortName=Params
  Bus Element Out1 : Outport  PortName=_Params

== system hodumaru/NeuralProcessingUnit/MiniColumn(Array)/MiniColumn1/Neuron(Array)/Neuron1/Soma/Membrane Potential Computing Unit ==
  Bus Element In4 : Inport  PortName=W_EN
  Bus Element In3 : Inport  Port=2  PortName=Spike Interval
  Bus Element In2 : Inport  Port=3  PortName=_Params
  Bus Element In1 : Inport  Port=4  PortName=Weight
  Bus Element Out2 : Outport  PortName=wait
  Bus Element Out1 : Outport  Port=2  PortName=Post Spike

== system hodumaru/NeuralProcessingUnit/MiniColumn(Array)/MiniColumn1/Neuron(Array)/Neuron1/Synapse/MUX ==
  Bus Element In3 : Inport  PortName=Control(R_EN)
  Bus Element In2 : Inport  Port=2  PortName=Control(Kill)
  Bus Element In1 : Inport  Port=3  PortName=R_DataOfSynapse
  Bus Element Out1 : Outport  PortName=TO_AXI
  Bus Element Out2 : Outport  Port=2  PortName=TO_INTERNAL

== system hodumaru/NeuralProcessingUnit/MiniColumn(Array)/MiniColumn1/Neuron(Array)/Neuron1/Synapse/Weight Table ==
  Bus Element In3 : Inport  PortName=W_EN
  Bus Element In5 : Inport  Port=2  PortName=R_EN_SY
  Bus Element In2 : Inport  Port=3  PortName=Data2Synapse
  Bus Element In1 : Inport  Port=4  PortName=Neuron ADDR
  Bus Element Out1 : Outport  PortName=R_DataOfSynapse
